simulink model "pfb_coeff_sim"  (R2016b)
settings: Solver=VariableStepAuto  StartTime=0.0  StopTime=8192*0.5  RelTol=1e-3
undefined symbols (not defined in the file): fft_stages
libraries: xbsIndex_r4 x6420, casper_library_misc x5, casper_library_sources x4, xps_library x1, casper_library_delays x1
(part 18 of 36)

== system pfb_coeff_sim/pfb/pfb_fir_generic/pfb_fir_coeff_gen ==
  sync : Inport
  din : Inport  Port=2
  en : Inport  Port=3
  a_expand : Subsystem  AncestorBlock=casper_library_flow_control/bus_expand  mask(bus_expand){mode=divisions of equal size, outputNum=64, outputWidth=18, outputBinaryPt=0, outputArithmeticType=0, show_format=off, outputToWorkspace=off, variablePrefix=out, outputToModelAsWell=on}
      mask prompts: outputNum "Number of outputs:"; outputWidth "Output width:"; outputBinaryPt "Output binary point position:"; outputArithmeticType "Output arithmetic type (ufix=0, fix=1, bool=2):"; show_format "Print format string?"; outputToWorkspace "Output to workspace?"; variablePrefix "Variable name prefix:"; outputToModelAsWell "Output to model as well?"
      mask help:
      | Expands a 'bus' made using a bus_create or Xilinx
      | concat block.
      | The input will be divided into the specified number
      | of outputs with the specified arithmetic types.
      | Divisions are made from most significant bit.
      mask init: same as pfb_coeff_sim/bus_expand5
      settings: AttributesFormatString=64 outputs
      mask TypeOptions mode: divisions of equal size | divisions of arbitrary size
      mask Callback mode: bus_expand_callback();
      mask Callback outputWidth: bus_expand_callback();
      mask Callback outputToWorkspace: bus_expand_callback();
  b_expand : Subsystem  AncestorBlock=casper_library_flow_control/bus_expand  mask(bus_expand){mode=divisions of equal size, outputNum=64, outputWidth=18, outputBinaryPt=0, outputArithmeticType=0, show_format=off, outputToWorkspace=off, variablePrefix=out, outputToModelAsWell=on}
      mask prompts: outputNum "Number of outputs:"; outputWidth "Output width:"; outputBinaryPt "Output binary point position:"; outputArithmeticType "Output arithmetic type (ufix=0, fix=1, bool=2):"; show_format "Print format string?"; outputToWorkspace "Output to workspace?"; variablePrefix "Variable name prefix:"; outputToModelAsWell "Output to model as well?"
      mask help:
      | Expands a 'bus' made using a bus_create or Xilinx
      | concat block.
      | The input will be divided into the specified number
      | of outputs with the specified arithmetic types.
      | Divisions are made from most significant bit.
      mask init: same as pfb_coeff_sim/bus_expand5
      settings: AttributesFormatString=64 outputs
      mask TypeOptions mode: divisions of equal size | divisions of arbitrary size
      mask Callback mode: bus_expand_callback();
      mask Callback outputWidth: bus_expand_callback();
      mask Callback outputToWorkspace: bus_expand_callback();
  concat : xbsIndex_r4/Concat  num_inputs=128  dbl_ovrd=off  block_type=concat
  const0 : xbsIndex_r4/Constant  const=1  gui_display_data_type=Fixed-point  arith_type=Signed (2's comp)  n_bits=18  bin_pt=17  preci_type=Single  exp_width=8  frac_width=24  explicit_period=on  period=1  equ=P=C  opselect=C  inp2=PCIN>>17  opr=+  inp1=P  carry=CIN  dbl_ovrd=off  block_type=constant
  const1 : xbsIndex_r4/Constant  const=3.7497e-17  gui_display_data_type=Fixed-point  arith_type=Signed (2's comp)  n_bits=18  bin_pt=17  preci_type=Single  exp_width=8  frac_width=24  explicit_period=on  period=1  equ=P=C  opselect=C  inp2=PCIN>>17  opr=+  inp1=P  carry=CIN  dbl_ovrd=off  block_type=constant
  const2 : xbsIndex_r4/Constant  const=-3.3271e-17  gui_display_data_type=Fixed-point  arith_type=Signed (2's comp)  n_bits=18  bin_pt=17  preci_type=Single  exp_width=8  frac_width=24  explicit_period=on  period=1  equ=P=C  opselect=C  inp2=PCIN>>17  opr=+  inp1=P  carry=CIN  dbl_ovrd=off  block_type=constant
  const3 : xbsIndex_r4/Constant  const=2.6947e-17  gui_display_data_type=Fixed-point  arith_type=Signed (2's comp)  n_bits=18  bin_pt=17  preci_type=Single  exp_width=8  frac_width=24  explicit_period=on  period=1  equ=P=C  opselect=C  inp2=PCIN>>17  opr=+  inp1=P  carry=CIN  dbl_ovrd=off  block_type=constant
  const4 : xbsIndex_r4/Constant  const=-1.9488e-17  gui_display_data_type=Fixed-point  arith_type=Signed (2's comp)  n_bits=18  bin_pt=17  preci_type=Single  exp_width=8  frac_width=24  explicit_period=on  period=1  equ=P=C  opselect=C  inp2=PCIN>>17  opr=+  inp1=P  carry=CIN  dbl_ovrd=off  block_type=constant
  const5 : xbsIndex_r4/Constant  const=1.2029e-17  gui_display_data_type=Fixed-point  arith_type=Signed (2's comp)  n_bits=18  bin_pt=17  preci_type=Single  exp_width=8  frac_width=24  explicit_period=on  period=1  equ=P=C  opselect=C  inp2=PCIN>>17  opr=+  inp1=P  carry=CIN  dbl_ovrd=off  block_type=constant
  const6 : xbsIndex_r4/Constant  const=-5.7064e-18  gui_display_data_type=Fixed-point  arith_type=Signed (2's comp)  n_bits=18  bin_pt=17  preci_type=Single  exp_width=8  frac_width=24  explicit_period=on  period=1  equ=P=C  opselect=C  inp2=PCIN>>17  opr=+  inp1=P  carry=CIN  dbl_ovrd=off  block_type=constant
  const7 : xbsIndex_r4/Constant  const=1.4823e-18  gui_display_data_type=Fixed-point  arith_type=Signed (2's comp)  n_bits=18  bin_pt=17  preci_type=Single  exp_width=8  frac_width=24  explicit_period=on  period=1  equ=P=C  opselect=C  inp2=PCIN>>17  opr=+  inp1=P  carry=CIN  dbl_ovrd=off  block_type=constant
  counter : xbsIndex_r4/Counter  cnt_type=Free Running  cnt_to=Inf  operation=Up  start_count=0  cnt_by_val=1  arith_type=Unsigned  n_bits=8  bin_pt=0  load_pin=off  rst=on  en=on  explicit_period=on  period=1  use_behavioral_HDL=off  implementation=Fabric  dbl_ovrd=off  block_type=counter
  d{0..63,65..71,73..79,81..87,89..95,97..103,105..111,113..119,121..127} (120 alike) : xbsIndex_r4/Delay  rst=off  infoeditControl=Selection of Reset will increase slice count due to use of real FFs and instead of SRLs  en=off  latency=1  reg_retiming=on  dbl_ovrd=off  block_type=delay
      settings: infoedit=Hardware notes: A delay line is a chain, each link of which is an SRL16 or SRL32 followed by a flip-flop.
  d{64,72,80,88,96,104,112,120} (8 alike) : xbsIndex_r4/Delay  rst=off  infoeditControl=Selection of Reset will increase slice count due to use of real FFs and instead of SRLs  en=on  latency=1  reg_retiming=on  dbl_ovrd=off  block_type=delay
      settings: infoedit=Hardware notes: A delay line is a chain, each link of which is an SRL16 or SRL32 followed by a flip-flop.
  den0 : xbsIndex_r4/Delay  rst=off  infoeditControl=Selection of Reset will increase slice count due to use of real FFs and instead of SRLs  en=off  latency=9  reg_retiming=on  dbl_ovrd=off  block_type=delay
      settings: infoedit=Hardware notes: A delay line is a chain, each link of which is an SRL16 or SRL32 followed by a flip-flop.
  den1 : xbsIndex_r4/Delay  rst=off  infoeditControl=Selection of Reset will increase slice count due to use of real FFs and instead of SRLs  en=off  latency=1  reg_retiming=on  dbl_ovrd=off  block_type=delay
      settings: infoedit=Hardware notes: A delay line is a chain, each link of which is an SRL16 or SRL32 followed by a flip-flop.
  dfirst : xbsIndex_r4/Delay  rst=off  infoeditControl=Selection of Reset will increase slice count due to use of real FFs and instead of SRLs  en=off  latency=3  reg_retiming=on  dbl_ovrd=off  block_type=delay
      settings: infoedit=Hardware notes: A delay line is a chain, each link of which is an SRL16 or SRL32 followed by a flip-flop.
  din_delay : xbsIndex_r4/Delay  rst=off  infoeditControl=Selection of Reset will increase slice count due to use of real FFs and instead of SRLs  en=off  latency=10  reg_retiming=on  dbl_ovrd=off  block_type=delay
      settings: infoedit=Hardware notes: A delay line is a chain, each link of which is an SRL16 or SRL32 followed by a flip-flop.
  first : xbsIndex_r4/Relational  mode=a=b  op_type=Bool  en=off  latency=6  dbl_ovrd=off  block_type=relational
  inverter : xbsIndex_r4/Inverter  en=off  latency=0  dbl_ovrd=off  block_type=inv
  munge : Subsystem  AncestorBlock=casper_library_flow_control/munge  mask(munge){divisions=64, div_size=[18 18 18 18 18 18 18 18 18 18 18 18 18 18 18 18 18 18 18 18 18 18 18 18 18 18 18 18 18 18 18 18 18 18 18 18 18 18 18 18 18 18 18 18 18 18 18 18 18 18 18 18 18 18 18 18 18 18 18 18 18 18 18 18], order=[56 63 62 61 60 59 58 57 48 55 54 53 52 51 50 49 40 47 46 45 44 43 42 41 32 39 38 37 36 35 34 33 24 31 30 29 28 27 26 25 16 23 22 21 20 19 18 17 8 15 14 13 12 11 10 9 0 7 6 5 4 3 2 1], arith_type_out=Unsigned, bin_pt_out=0}
      mask prompts: divisions "Number of divisions"; div_size "Division size (bits)"; order "Division packing order"; arith_type_out "Output arithmetic type"; bin_pt_out "Output binary point"
      mask help: Splits an input bus into the specified number of divisions and then recombines them in the order specified (most significant division = 0,least = number divisions-1)
      mask init:
      | munge_init(gcb, ...
      |     'divisions', divisions, ...
      |     'div_size', div_size, ...
      |     'order', order, ...
      |     'arith_type_out', arith_type_out, ...
      |     'bin_pt_out', bin_pt_out);
      settings: AttributesFormatString=|
      | split:[18 18 18 18 18 18 18 18 18 18 18 18 18 18 18 18 18 18 18 18 18 18 18 18 18 18 18 18 18 18 18 18 18 18 18 18 18 18 18 18 18 18 18 18 18 18 18 18 18 18 18 18 18 18 18 18 18 18 18 18 18 18 18 18]
      | join:[56 63 62 61 60 59 58 57 48 55 54 53 52 51 50 49 40 47 46 45 44 43 42 41 32 39 38 37 36 35 34 33 24 31 30 29 28 27 26 25 16 23 22 21 20 19 18 17 8 15 14 13 12 11 10 9 0 7 6 5 4 3 2 1]
      | Unsigned [1152,0]
      mask TypeOptions arith_type_out: Unsigned | Signed  (2's comp) | Floating-point
  mux{0..7} (8 alike) : xbsIndex_r4/Mux  inputs=2  en=off  latency=1  precision=Full  arith_type=Unsigned  n_bits=16  bin_pt=14  quantization=Truncate  overflow=Wrap  dbl_ovrd=off  block_type=mux
  reinterpret{0..7} (8 alike) : xbsIndex_r4/Reinterpret  force_arith_type=on  arith_type=Unsigned  force_bin_pt=on  bin_pt=0  block_type=reinterpret
  rom : Subsystem  AncestorBlock=casper_library_bus/bus_dual_port_ram  mask(bus_dual_port_ram){n_bits=[18 18 18 18 18 18 18 18 18 18 18 18 18 18 18 18 18 18 18 18 18 18 18 18 18 18 18 18 18 18 18 18 18 18 18 18 18 18 18 18 18 18 18 18 18 18 18 18 18 18 18 18 18 18 18 18 18 18 18 18 18 18 18 18], bin_pts=[17 17 17 17 17 17 17 17 17 17 17 17 17 17 17 17 17 17 17 17 17 17 17 17 17 17 17 17 17 17 17 17 17 17 17 17 17 17 17 17 17 17 17 17 17 17 17 17 17 17 17 17 17 17 17 17 17 17 17 17 17 17 17 17], init_vector=[pfb_coeff_gen_calc(11, 16, 'hann', 3, 0, 1, 1, false)', pfb_coeff_gen_calc(11, 16, 'hann', 3, 1, 1, 1, false)', pfb_coeff_gen_calc(11, 16, 'hann', 3, 2, 1, 1, false)', pfb_coeff_gen_calc(11, 16, 'hann', 3, 3, 1, 1, false)', pfb_coeff_gen_calc(11, 16, 'hann', 3, 4, 1, 1, false)', pfb_coeff_gen_calc(11, 16, 'hann', 3, 5, 1, 1, false)', pfb_coeff_gen_calc(11, 16, 'hann', 3, 6, 1, 1, false)', pfb_coeff_gen_calc(11, 16, 'hann', 3, 7, 1, 1, false)', pfb_coeff_gen_calc(11, 16, 'hann', 3, 0, 1, 2, false)', pfb_coeff_gen_calc(11, 16, 'hann', 3, 1, 1, 2, false)', pfb_coeff_gen_calc(11, 16, 'hann', 3, 2, 1, 2, false)', pfb_coeff_gen_calc(11, 16, 'hann', 3, 3, 1, 2, false)', pfb_coeff_gen_calc(11, 16, 'hann', 3, 4, 1, 2, false)', pfb_coeff_gen_calc(11, 16, 'hann', 3, 5, 1, 2, false)', pfb_coeff_gen_calc(11, 16, 'hann', 3, 6, 1, 2, false)', pfb_coeff_gen_calc(11, 16, 'hann', 3, 7, 1, 2, false)', pfb_coeff_gen_calc(11, 16, 'hann', 3, 0, 1, 3, false)', pfb_coeff_gen_calc(11, 16, 'hann', 3, 1, 1, 3, false)', pfb_coeff_gen_calc(11, 16, 'hann', 3, 2, 1, 3, false)', pfb_coeff_gen_calc(11, 16, 'hann', 3, 3, 1, 3, false)', pfb_coeff_gen_calc(11, 16, 'hann', 3, 4, 1, 3, false)', pfb_coeff_gen_calc(11, 16, 'hann', 3, 5, 1, 3, false)', pfb_coeff_gen_calc(11, 16, 'hann', 3, 6, 1, 3, false)', pfb_coeff_gen_calc(11, 16, 'hann', 3, 7, 1, 3, false)', pfb_coeff_gen_calc(11, 16, 'hann', 3, 0, 1, 4, false)', pfb_coeff_gen_calc(11, 16, 'hann', 3, 1, 1, 4, false)', pfb_coeff_gen_calc(11, 16, 'hann', 3, 2, 1, 4, false)', pfb_coeff_gen_calc(11, 16, 'hann', 3, 3, 1, 4, false)', pfb_coeff_gen_calc(11, 16, 'hann', 3, 4, 1, 4, false)', pfb_coeff_gen_calc(11, 16, 'hann', 3, 5, 1, 4, false)', pfb_coeff_gen_calc(11, 16, 'hann', 3, 6, 1, 4, false)', pfb_coeff_gen_calc(11, 16, 'hann', 3, 7, 1, 4, false)', pfb_coeff_gen_calc(11, 16, 'hann', 3, 0, 1, 5, false)', pfb_coeff_gen_calc(11, 16, 'hann', 3, 1, 1, 5, false)', pfb_coeff_gen_calc(11, 16, 'hann', 3, 2, 1, 5, false)', pfb_coeff_gen_calc(11, 16, 'hann', 3, 3, 1, 5, false)', pfb_coeff_gen_calc(11, 16, 'hann', 3, 4, 1, 5, false)', pfb_coeff_gen_calc(11, 16, 'hann', 3, 5, 1, 5, false)', pfb_coeff_gen_calc(11, 16, 'hann', 3, 6, 1, 5, false)', pfb_coeff_gen_calc(11, 16, 'hann', 3, 7, 1, 5, false)', pfb_coeff_gen_calc(11, 16, 'hann', 3, 0, 1, 6, false)', pfb_coeff_gen_calc(11, 16, 'hann', 3, 1, 1, 6, false)', pfb_coeff_gen_calc(11, 16, 'hann', 3, 2, 1, 6, false)', pfb_coeff_gen_calc(11, 16, 'hann', 3, 3, 1, 6, false)', pfb_coeff_gen_calc(11, 16, 'hann', 3, 4, 1, 6, false)', pfb_coeff_gen_calc(11, 16, 'hann', 3, 5, 1, 6, false)', pfb_coeff_gen_calc(11, 16, 'hann', 3, 6, 1, 6, false)', pfb_coeff_gen_calc(11, 16, 'hann', 3, 7, 1, 6, false)', pfb_coeff_gen_calc(11, 16, 'hann', 3, 0, 1, 7, false)', pfb_coeff_gen_calc(11, 16, 'hann', 3, 1, 1, 7, false)', pfb_coeff_gen_calc(11, 16, 'hann', 3, 2, 1, 7, false)', pfb_coeff_gen_calc(11, 16, 'hann', 3, 3, 1, 7, false)', pfb_coeff_gen_calc(11, 16, 'hann', 3, 4, 1, 7, false)', pfb_coeff_gen_calc(11, 16, 'hann', 3, 5, 1, 7, false)', pfb_coeff_gen_calc(11, 16, 'hann', 3, 6, 1, 7, false)', pfb_coeff_gen_calc(11, 16, 'hann', 3, 7, 1, 7, false)', pfb_coeff_gen_calc(11, 16, 'hann', 3, 0, 1, 8, false)', pfb_coeff_gen_calc(11, 16, 'hann', 3, 1, 1, 8, false)', pfb_coeff_gen_calc(11, 16, 'hann', 3, 2, 1, 8, false)', pfb_coeff_gen_calc(11, 16, 'hann', 3, 3, 1, 8, false)', pfb_coeff_gen_calc(11, 16, 'hann', 3, 4, 1, 8, false)', pfb_coeff_gen_calc(11, 16, 'hann', 3, 5, 1, 8, false)', pfb_coeff_gen_calc(11, 16, 'hann', 3, 6, 1, 8, false)', pfb_coeff_gen_calc(11, 16, 'hann', 3, 7, 1, 8, false)'], max_fanout=1, mem_type=Block RAM, bram_optimization=Speed, async_a=off, async_b=off, b_to_a_ratio_bits=0, misc=off, bram_latency=3, fan_latency=6, addra_register=on, addra_implementation=core, dina_register=off, dina_implementation=behavioral, wea_register=off, wea_implementation=behavioral, ena_register=off, ena_implementation=core, addrb_register=on, addrb_implementation=core, dinb_register=off, dinb_implementation=behavioral, web_register=off, web_implementation=behavioral, enb_register=off, enb_implementation=core}
      mask prompts: n_bits "data word bit widths"; bin_pts "data word binary points"; init_vector "initial value vector"; max_fanout "limit fanout to ?"; mem_type "memory type"; bram_optimization "memory optimization"; async_a "a asynchronous"; async_b "b asynchronous"; b_to_a_ratio_bits "b_to_a ratio bits"; misc "misc support"; bram_latency "bram latency"; fan_latency "input register latency"; addra_register "addra input register"; addra_implementation "addra register implementation"; dina_register "dina input register"; dina_implementation "dina register implementation"; wea_register "wea input register"; wea_implementation "wea register implementation"; ena_register "ena input register"; ena_implementation "ena register implementation"; addrb_register "addrb input register"; addrb_implementation "addrb register implementation"; dinb_register "dinb input register"; dinb_implementation "dinb register implementation"; web_register "web input register"; web_implementation "web register implementation"; enb_register "enb input register"; enb_implementation "enb register implementation"
      mask help: RAM for a bus allowing fanout control
      mask init:
      | bus_dual_port_ram_init(gcb, ...
      |     'n_bits', n_bits, ...
      |     'bin_pts', bin_pts, ...
      |     'init_vector', init_vector, ...
      |     'max_fanout', max_fanout, ...
      |     'mem_type', mem_type, ...
      |     'bram_optimization', bram_optimization, ...
      |     'async_a', async_a, ...
      |     'async_b', async_b, ...
      |     'b_to_a_ratio_bits', b_to_a_ratio_bits, ...
      |     'misc', misc, ...
      |     'bram_latency', bram_latency, ...
      |     'fan_latency', fan_latency, ...
      |     'addra_register', addra_register, ...
      |     'addra_implementation', addra_implementation, ...
      |     'dina_register', dina_register, ...
      |     'dina_implementation', dina_implementation, ...
      |     'wea_register', wea_register, ...
      |     'wea_implementation', wea_implementation, ...
      |     'ena_register', ena_register, ...
      |     'ena_implementation', ena_implementation, ...
      |     'addrb_register', addrb_register, ...
      |     'addrb_implementation', addrb_implementation, ...
      |     'dinb_register', dinb_register, ...
      |     'dinb_implementation', dinb_implementation, ...
      |     'web_register', web_register, ...
      |     'web_implementation', web_implementation, ...
      |     'enb_register', enb_register, ...
      |     'enb_implementation', enb_implementation);
      mask TypeOptions mem_type: Distributed memory | Block RAM
      mask TypeOptions bram_optimization: Area | Speed
      mask TypeOptions addra_implementation: core | behavioral
      mask TypeOptions dina_implementation: core | behavioral
      mask TypeOptions wea_implementation: core | behavioral
      mask TypeOptions ena_implementation: core | behavioral
      mask TypeOptions addrb_implementation: core | behavioral
      mask TypeOptions dinb_implementation: core | behavioral
      mask TypeOptions web_implementation: core | behavioral
      mask TypeOptions enb_implementation: core | behavioral
  rom_din : xbsIndex_r4/Constant  const=0  gui_display_data_type=Fixed-point  arith_type=Unsigned  n_bits=1152  bin_pt=0  preci_type=Single  exp_width=8  frac_width=24  explicit_period=on  period=1  equ=P=C  opselect=C  inp2=PCIN>>17  opr=+  inp1=P  carry=CIN  dbl_ovrd=off  block_type=constant
  rom_we : xbsIndex_r4/Constant  const=0  gui_display_data_type=Fixed-point  arith_type=Boolean  n_bits=16  bin_pt=14  preci_type=Single  exp_width=8  frac_width=24  explicit_period=on  period=1  equ=P=C  opselect=C  inp2=PCIN>>17  opr=+  inp1=P  carry=CIN  dbl_ovrd=off  block_type=constant
  sync_delay : xbsIndex_r4/Delay  rst=off  infoeditControl=Selection of Reset will increase slice count due to use of real FFs and instead of SRLs  en=off  latency=10  reg_retiming=on  dbl_ovrd=off  block_type=delay
      settings: infoedit=Hardware notes: A delay line is a chain, each link of which is an SRL16 or SRL32 followed by a flip-flop.
  zero : xbsIndex_r4/Constant  const=0  gui_display_data_type=Fixed-point  arith_type=Unsigned  n_bits=8  bin_pt=0  preci_type=Single  exp_width=8  frac_width=24  explicit_period=on  period=1  equ=P=C  opselect=C  inp2=PCIN>>17  opr=+  inp1=P  carry=CIN  dbl_ovrd=off  block_type=constant
  sync_out : Outport
  dout : Outport  Port=2
  coeffs : Outport  Port=3
  dvalid : Outport  Port=4
  wires:
  sync/1 -> sync_delay/1, counter/1
  sync_delay/1 -> sync_out/1
  din/1 -> din_delay/1
  din_delay/1 -> dout/1
  counter/1 -> inverter/1, rom/1(addra), first/2
  inverter/1 -> rom/4(addrb)
  rom_din/1 -> rom/2(dina), rom/5(dinb)
  rom_we/1 -> rom/3(wea), rom/6(web)
  zero/1 -> first/1
  first/1 -> dfirst/1
  rom/2(B) -> munge/1(din)
  rom/1(A) -> a_expand/1(bus_in)
  munge/1(dout) -> b_expand/1(bus_in)
  concat/1 -> coeffs/1
  a_expand/1(msb_out64) -> d0/1
  d0/1 -> concat/1
  a_expand/2(out63) -> d1/1
  d1/1 -> concat/2
  a_expand/3(out62) -> d2/1
  d2/1 -> concat/3
  a_expand/4(out61) -> d3/1
  d3/1 -> concat/4
  a_expand/5(out60) -> d4/1
  d4/1 -> concat/5
  a_expand/6(out59) -> d5/1
  d5/1 -> concat/6
  a_expand/7(out58) -> d6/1
  d6/1 -> concat/7
  a_expand/8(out57) -> d7/1
  d7/1 -> concat/8
  a_expand/9(out56) -> d8/1
  d8/1 -> concat/9
  a_expand/10(out55) -> d9/1
  d9/1 -> concat/10
  a_expand/11(out54) -> d10/1
  d10/1 -> concat/11
  a_expand/12(out53) -> d11/1
  d11/1 -> concat/12
  a_expand/13(out52) -> d12/1
  d12/1 -> concat/13
  a_expand/14(out51) -> d13/1
  d13/1 -> concat/14
  a_expand/15(out50) -> d14/1
  d14/1 -> concat/15
  a_expand/16(out49) -> d15/1
  d15/1 -> concat/16
  a_expand/17(out48) -> d16/1
  d16/1 -> concat/17
  a_expand/18(out47) -> d17/1
  d17/1 -> concat/18
  a_expand/19(out46) -> d18/1
  d18/1 -> concat/19
  a_expand/20(out45) -> d19/1
  d19/1 -> concat/20
  a_expand/21(out44) -> d20/1
  d20/1 -> concat/21
  a_expand/22(out43) -> d21/1
  d21/1 -> concat/22
  a_expand/23(out42) -> d22/1
  d22/1 -> concat/23
  a_expand/24(out41) -> d23/1
  d23/1 -> concat/24
  a_expand/25(out40) -> d24/1
  d24/1 -> concat/25
  a_expand/26(out39) -> d25/1
  d25/1 -> concat/26
  a_expand/27(out38) -> d26/1
  d26/1 -> concat/27
  a_expand/28(out37) -> d27/1
  d27/1 -> concat/28
  a_expand/29(out36) -> d28/1
  d28/1 -> concat/29
  a_expand/30(out35) -> d29/1
  d29/1 -> concat/30
  a_expand/31(out34) -> d30/1
  d30/1 -> concat/31
  a_expand/32(out33) -> d31/1
  d31/1 -> concat/32
  a_expand/33(out32) -> d32/1
  d32/1 -> concat/33
  a_expand/34(out31) -> d33/1
  d33/1 -> concat/34
  a_expand/35(out30) -> d34/1
  d34/1 -> concat/35
  a_expand/36(out29) -> d35/1
  d35/1 -> concat/36
  a_expand/37(out28) -> d36/1
  d36/1 -> concat/37
  a_expand/38(out27) -> d37/1
  d37/1 -> concat/38
  a_expand/39(out26) -> d38/1
  d38/1 -> concat/39
  a_expand/40(out25) -> d39/1
  d39/1 -> concat/40
  a_expand/41(out24) -> d40/1
  d40/1 -> concat/41
  a_expand/42(out23) -> d41/1
  d41/1 -> concat/42
  a_expand/43(out22) -> d42/1
  d42/1 -> concat/43
  a_expand/44(out21) -> d43/1
  d43/1 -> concat/44
  a_expand/45(out20) -> d44/1
  d44/1 -> concat/45
  a_expand/46(out19) -> d45/1
  d45/1 -> concat/46
  a_expand/47(out18) -> d46/1
  d46/1 -> concat/47
  a_expand/48(out17) -> d47/1
  d47/1 -> concat/48
  a_expand/49(out16) -> d48/1
  d48/1 -> concat/49
  a_expand/50(out15) -> d49/1
  d49/1 -> concat/50
  a_expand/51(out14) -> d50/1
  d50/1 -> concat/51
  a_expand/52(out13) -> d51/1
  d51/1 -> concat/52
  a_expand/53(out12) -> d52/1
  d52/1 -> concat/53
  a_expand/54(out11) -> d53/1
  d53/1 -> concat/54
  a_expand/55(out10) -> d54/1
  d54/1 -> concat/55
  a_expand/56(out9) -> d55/1
  d55/1 -> concat/56
  a_expand/57(out8) -> d56/1
  d56/1 -> concat/57
  a_expand/58(out7) -> d57/1
  d57/1 -> concat/58
  a_expand/59(out6) -> d58/1
  d58/1 -> concat/59
  a_expand/60(out5) -> d59/1
  d59/1 -> concat/60
  a_expand/61(out4) -> d60/1
  d60/1 -> concat/61
  a_expand/62(out3) -> d61/1
  d61/1 -> concat/62
  a_expand/63(out2) -> d62/1
  d62/1 -> concat/63
  a_expand/64(lsb_out1) -> d63/1
  d63/1 -> concat/64
  b_expand/1(msb_out64) -> d64/1
  const0/1 -> reinterpret0/1
  reinterpret0/1 -> mux0/3
  dfirst/1 -> mux0/1, mux1/1, mux2/1, mux3/1, mux4/1, mux5/1, mux6/1, mux7/1
  d64/1 -> mux0/2
  mux0/1 -> concat/65
  b_expand/2(out63) -> d65/1
  d65/1 -> concat/66
  b_expand/3(out62) -> d66/1
  d66/1 -> concat/67
  b_expand/4(out61) -> d67/1
  d67/1 -> concat/68
  b_expand/5(out60) -> d68/1
  d68/1 -> concat/69
  b_expand/6(out59) -> d69/1
  d69/1 -> concat/70
  b_expand/7(out58) -> d70/1
  d70/1 -> concat/71
  b_expand/8(out57) -> d71/1
  d71/1 -> concat/72
  b_expand/9(out56) -> d72/1
  const1/1 -> reinterpret1/1
  reinterpret1/1 -> mux1/3
  d72/1 -> mux1/2
  mux1/1 -> concat/73
  b_expand/10(out55) -> d73/1
  d73/1 -> concat/74
  b_expand/11(out54) -> d74/1
  d74/1 -> concat/75
  b_expand/12(out53) -> d75/1
  d75/1 -> concat/76
  b_expand/13(out52) -> d76/1
  d76/1 -> concat/77
  b_expand/14(out51) -> d77/1
  d77/1 -> concat/78
  b_expand/15(out50) -> d78/1
  d78/1 -> concat/79
  b_expand/16(out49) -> d79/1
  d79/1 -> concat/80
  b_expand/17(out48) -> d80/1
  const2/1 -> reinterpret2/1
  reinterpret2/1 -> mux2/3
  d80/1 -> mux2/2
  mux2/1 -> concat/81
  b_expand/18(out47) -> d81/1
  d81/1 -> concat/82
  b_expand/19(out46) -> d82/1
  d82/1 -> concat/83
  b_expand/20(out45) -> d83/1
  d83/1 -> concat/84
  b_expand/21(out44) -> d84/1
  d84/1 -> concat/85
  b_expand/22(out43) -> d85/1
  d85/1 -> concat/86
  b_expand/23(out42) -> d86/1
  d86/1 -> concat/87
  b_expand/24(out41) -> d87/1
  d87/1 -> concat/88
  b_expand/25(out40) -> d88/1
  const3/1 -> reinterpret3/1
  reinterpret3/1 -> mux3/3
  d88/1 -> mux3/2
  mux3/1 -> concat/89
  b_expand/26(out39) -> d89/1
  d89/1 -> concat/90
  b_expand/27(out38) -> d90/1
  d90/1 -> concat/91
  b_expand/28(out37) -> d91/1
  d91/1 -> concat/92
  b_expand/29(out36) -> d92/1
  d92/1 -> concat/93
  b_expand/30(out35) -> d93/1
  d93/1 -> concat/94
  b_expand/31(out34) -> d94/1
  d94/1 -> concat/95
  b_expand/32(out33) -> d95/1
  d95/1 -> concat/96
  b_expand/33(out32) -> d96/1
  const4/1 -> reinterpret4/1
  reinterpret4/1 -> mux4/3
  d96/1 -> mux4/2
  mux4/1 -> concat/97
  b_expand/34(out31) -> d97/1
  d97/1 -> concat/98
  b_expand/35(out30) -> d98/1
  d98/1 -> concat/99
  b_expand/36(out29) -> d99/1
  d99/1 -> concat/100
  b_expand/37(out28) -> d100/1
  d100/1 -> concat/101
  b_expand/38(out27) -> d101/1
  d101/1 -> concat/102
  b_expand/39(out26) -> d102/1
  d102/1 -> concat/103
  b_expand/40(out25) -> d103/1
  d103/1 -> concat/104
  b_expand/41(out24) -> d104/1
  const5/1 -> reinterpret5/1
  reinterpret5/1 -> mux5/3
  d104/1 -> mux5/2
  mux5/1 -> concat/105
  b_expand/42(out23) -> d105/1
  d105/1 -> concat/106
  b_expand/43(out22) -> d106/1
  d106/1 -> concat/107
  b_expand/44(out21) -> d107/1
  d107/1 -> concat/108
  b_expand/45(out20) -> d108/1
  d108/1 -> concat/109
  b_expand/46(out19) -> d109/1
  d109/1 -> concat/110
  b_expand/47(out18) -> d110/1
  d110/1 -> concat/111
  b_expand/48(out17) -> d111/1
  d111/1 -> concat/112
  b_expand/49(out16) -> d112/1
  const6/1 -> reinterpret6/1
  reinterpret6/1 -> mux6/3
  d112/1 -> mux6/2
  mux6/1 -> concat/113
  b_expand/50(out15) -> d113/1
  d113/1 -> concat/114
  b_expand/51(out14) -> d114/1
  d114/1 -> concat/115
  b_expand/52(out13) -> d115/1
  d115/1 -> concat/116
  b_expand/53(out12) -> d116/1
  d116/1 -> concat/117
  b_expand/54(out11) -> d117/1
  d117/1 -> concat/118
  b_expand/55(out10) -> d118/1
  d118/1 -> concat/119
  b_expand/56(out9) -> d119/1
  d119/1 -> concat/120
  b_expand/57(out8) -> d120/1
  const7/1 -> reinterpret7/1
  reinterpret7/1 -> mux7/3
  d120/1 -> mux7/2
  mux7/1 -> concat/121
  b_expand/58(out7) -> d121/1
  d121/1 -> concat/122
  b_expand/59(out6) -> d122/1
  d122/1 -> concat/123
  b_expand/60(out5) -> d123/1
  d123/1 -> concat/124
  b_expand/61(out4) -> d124/1
  d124/1 -> concat/125
  b_expand/62(out3) -> d125/1
  d125/1 -> concat/126
  b_expand/63(out2) -> d126/1
  d126/1 -> concat/127
  b_expand/64(lsb_out1) -> d127/1
  d127/1 -> concat/128
  en/1 -> counter/2, den0/1
  den0/1 -> d64/2, d72/2, d80/2, d88/2, d96/2, d104/2, d112/2, d120/2, den1/1
  den1/1 -> dvalid/1

== system pfb_coeff_sim/pfb/pfb_fir_generic/pfb_fir_taps ==
  sync : Inport
  din : Inport  Port=2
  coeffs : Inport  Port=3
  en : Inport  Port=4
  arnold : Terminator
  bram_din : xbsIndex_r4/Concat  num_inputs=2  dbl_ovrd=off  block_type=concat
  bus_adder_tree : Subsystem  AncestorBlock=casper_library_bus/bus_adder_tree  mask(bus_adder_tree){n_busses=16, n_bits=[28 28 28 28 28 28 28 28], bin_pts=26, dtypes=1, add_latency=4, first_stage_hdl=on, adder_imp=Behavioral, misc=off}
      mask prompts: n_busses "number of busses"; n_bits "bus component bit widths"; bin_pts "bus component binary points"; dtypes "bus component data types"; add_latency "adder latency"; first_stage_hdl "implement first stage in of adders in behavioral HDL?"; adder_imp "adder implementation"; misc "misc support"
      mask help: Add components of multiple identical busses
      mask init:
      | bus_adder_tree_init(gcb, ...
      |     'n_busses', n_busses, ...
      |     'n_bits', n_bits, ...
      |     'bin_pts', bin_pts, ...
      |     'dtypes', dtypes, ...
      |     'add_latency', add_latency, ...
      |     'first_stage_hdl', first_stage_hdl, ...
      |     'adder_imp', adder_imp, ...
      |     'misc', misc);
      mask TypeOptions adder_imp: Behavioral | Fabric | DSP48
  bus_mult : Subsystem  AncestorBlock=casper_library_bus/bus_mult  mask(bus_mult){n_bits_a=[10 10 10 10 10 10 10 10 10 10 10 10 10 10 10 10 10 10 10 10 10 10 10 10 10 10 10 10 10 10 10 10 10 10 10 10 10 10 10 10 10 10 10 10 10 10 10 10 10 10 10 10 10 10 10 10 10 10 10 10 10 10 10 10 10 10 10 10 10 10 10 10 10 10 10 10 10 10 10 10 10 10 10 10 10 10 10 10 10 10 10 10 10 10 10 10 10 10 10 10 10 10 10 10 10 10 10 10 10 10 10 10 10 10 10 10 10 10 10 10 10 10 10 10 10 10 10 10], bin_pt_a=9, type_a=1, cmplx_a=off, n_bits_b=[18 18 18 18 18 18 18 18 18 18 18 18 18 18 18 18 18 18 18 18 18 18 18 18 18 18 18 18 18 18 18 18 18 18 18 18 18 18 18 18 18 18 18 18 18 18 18 18 18 18 18 18 18 18 18 18 18 18 18 18 18 18 18 18 18 18 18 18 18 18 18 18 18 18 18 18 18 18 18 18 18 18 18 18 18 18 18 18 18 18 18 18 18 18 18 18 18 18 18 18 18 18 18 18 18 18 18 18 18 18 18 18 18 18 18 18 18 18 18 18 18 18 18 18 18 18 18 18], bin_pt_b=17, type_b=1, cmplx_b=off, misc=off, floating_point=off, float_type=single, input_vec_a=1, input_vec_b=1, frac_width=19, exp_width=6, n_bits_out=n_bits_data+n_bits_coeff, bin_pt_out=n_bits_data-1+bin_pt_coeff, type_out=1, quantization=0, overflow=0, mult_latency=mult_latency, add_latency=0, conv_latency=0, max_fanout=1, fan_latency=0, multiplier_implementation=behavioral HDL, pipeline_cmult_en=off, pipeline_latency=0}
      mask prompts: n_bits_a "a input bit widths"; bin_pt_a "a input binary points"; type_a "a input type (Unsigned=0, Signed=1)"; cmplx_a "a input complex"; n_bits_b "b input bit widths"; bin_pt_b "b input binary points"; type_b "b input type (Unsigned=0, Signed=1)"; cmplx_b "b input complex"; misc "misc support"; floating_point "floating point"; float_type "float type"; input_vec_a "a input vector in bus"; input_vec_b "b input vector in bus"; frac_width "fraction width"; exp_width "exponent width"; n_bits_out "output bit widths"; bin_pt_out "output binary points"; type_out "output type (Unsigned=0, Signed=1)"; quantization "quantization strategy (Truncate=0, Round  (unbiased: +/- Inf)=1)"; overflow "overflow strategy (Wrap=0, Saturate=1, Flag as error=2)"; mult_latency "multiplier latency"; add_latency "adder latency"; conv_latency "convert latency"; max_fanout "limit fanout to ?"; fan_latency "fanout register latency"; multiplier_implementation "multiplier implementation"; pipeline_cmult_en "pipeline complex mult"; pipeline_latency "pipeline latency"
      mask help: Multiply components of two busses
      mask init:
      | bus_mult_init(gcb, ...
      |     'n_bits_a', n_bits_a, ...
      |     'bin_pt_a', bin_pt_a, ...
      |     'type_a', type_a, ...
      |     'cmplx_a', cmplx_a, ...
      |     'n_bits_b', n_bits_b, ...
      |     'bin_pt_b', bin_pt_b, ...
      |     'type_b', type_b, ...
      |     'cmplx_b', cmplx_b, ...
      |     'n_bits_out', n_bits_out, ...
      |     'bin_pt_out', bin_pt_out, ...
      |     'type_out', type_out, ...
      |     'floating_point', floating_point, ...
      |     'float_type', float_type, ...
      |     'exp_width', exp_width, ...
      |     'input_vec_a', input_vec_a, ...
      |     'input_vec_b', input_vec_b, ...
      |     'frac_width', frac_width, ...         
      |     'quantization', quantization, ...
      |     'overflow', overflow, ...
      |     'mult_latency', mult_latency, ...
      |     'add_latency', add_latency, ...
      |     'conv_latency', conv_latency, ...
      |     'max_fanout', max_fanout, ...
      |     'pipeline_cmult_en', pipeline_cmult_en, ...
      |     'pipeline_latency', pipeline_latency, ...
      |     'fan_latency', fan_latency, ...
      |     'multiplier_implementation', multiplier_implementation, ...
      |     'misc', misc);
      mask Callback floating_point:
      | onoff = get_param(gcb, 'floating_point');
      | if strcmp(onoff,'on')
      |     enable_fixpt = 'off'
      |     set_param_state(gcb, 'float_type', 'on')
      | 
      |     set_param_state(gcb, 'input_vec_a', 'on')
      |     set_param_state(gcb, 'input_vec_b', 'on')
      | 
      |     f_type = get_param(gcb, 'float_type')
      |     if strcmp(f_type,'custom')
      |         set_param_state(gcb, 'exp_width', 'on')
      |         set_param_state(gcb, 'frac_width', 'on')
      |     else
      |         set_param_state(gcb, 'exp_width', 'off')
      |         set_param_state(gcb, 'frac_width', 'off')
      |     end
      | 
      | else
      |     enable_fixpt = 'on'
      |     set_param_state(gcb, 'float_type', 'off')
      |     set_param_state(gcb, 'exp_width', 'off')
      |     set_param_state(gcb, 'frac_width', 'off')
      |     set_param_state(gcb, 'input_vec_a', 'off')
      |     set_param_state(gcb, 'input_vec_b', 'off')
      | end
      | 
      | set_param_state(gcb, 'n_bits_a', enable_fixpt)
      | set_param_state(gcb, 'bin_pt_a', enable_fixpt)
      | set_param_state(gcb, 'type_a', enable_fixpt)
      | set_param_state(gcb, 'n_bits_b', enable_fixpt)
      | set_param_state(gcb, 'bin_pt_b', enable_fixpt)
      | set_param_state(gcb, 'type_b', enable_fixpt)
      | 
      | set_param_state(gcb, 'n_bits_out', enable_fixpt)
      | set_param_state(gcb, 'bin_pt_out', enable_fixpt)
      | set_param_state(gcb, 'type_out', enable_fixpt)
      | set_param_state(gcb, 'quantization', enable_fixpt)
      | set_param_state(gcb, 'overflow', enable_fixpt)
      mask TypeOptions float_type: single | custom
      mask Callback float_type:
      | f_type = get_param(gcb, 'float_type')
      | if strcmp(f_type,'custom')
      |     set_param_state(gcb, 'exp_width', 'on')
      |     set_param_state(gcb, 'frac_width', 'on')
      | else
      |     set_param_state(gcb, 'exp_width', 'off')
      |     set_param_state(gcb, 'frac_width', 'off')
      | end
      mask TypeOptions multiplier_implementation: behavioral HDL | standard core | embedded multiplier core
      mask Callback pipeline_cmult_en:
      | pipeline_en = get_param(gcb, 'pipeline_cmult_en');
      | if strcmp(pipeline_en,'on')
      | 
      |     set_param_state(gcb, 'pipeline_latency', 'on')
      | else
      |     set_param_state(gcb, 'pipeline_latency', 'off')
      | end
  counter : xbsIndex_r4/Counter  cnt_type=Free Running  cnt_to=Inf  operation=Up  start_count=0  cnt_by_val=1  arith_type=Unsigned  n_bits=8  bin_pt=0  load_pin=off  rst=on  en=on  explicit_period=on  period=1  use_behavioral_HDL=off  implementation=Fabric  dbl_ovrd=off  block_type=counter
  daddr : xbsIndex_r4/Delay  rst=off  infoeditControl=Selection of Reset will increase slice count due to use of real FFs and instead of SRLs  en=off  latency=9  reg_retiming=on  dbl_ovrd=off  block_type=delay
      settings: infoedit=Hardware notes: A delay line is a chain, each link of which is an SRL16 or SRL32 followed by a flip-flop.
  dcoeffs : xbsIndex_r4/Delay  rst=off  infoeditControl=Selection of Reset will increase slice count due to use of real FFs and instead of SRLs  en=off  latency=9  reg_retiming=on  dbl_ovrd=off  block_type=delay
      settings: infoedit=Hardware notes: A delay line is a chain, each link of which is an SRL16 or SRL32 followed by a flip-flop.
  ddin : xbsIndex_r4/Delay  rst=off  infoeditControl=Selection of Reset will increase slice count due to use of real FFs and instead of SRLs  en=off  latency=9  reg_retiming=off  dbl_ovrd=off  block_type=delay
      settings: infoedit=Hardware notes: A delay line is a chain, each link of which is an SRL16 or SRL32 followed by a flip-flop.
  den0 : xbsIndex_r4/Delay  rst=off  infoeditControl=Selection of Reset will increase slice count due to use of real FFs and instead of SRLs  en=off  latency=9  reg_retiming=on  dbl_ovrd=off  block_type=delay
      settings: infoedit=Hardware notes: A delay line is a chain, each link of which is an SRL16 or SRL32 followed by a flip-flop.
  den1 : xbsIndex_r4/Delay  rst=off  infoeditControl=Selection of Reset will increase slice count due to use of real FFs and instead of SRLs  en=off  latency=3  reg_retiming=on  dbl_ovrd=off  block_type=delay
      settings: infoedit=Hardware notes: A delay line is a chain, each link of which is an SRL16 or SRL32 followed by a flip-flop.
  den2 : xbsIndex_r4/Delay  rst=off  infoeditControl=Selection of Reset will increase slice count due to use of real FFs and instead of SRLs  en=off  latency=16  reg_retiming=on  dbl_ovrd=off  block_type=delay
      settings: infoedit=Hardware notes: A delay line is a chain, each link of which is an SRL16 or SRL32 followed by a flip-flop.
  dsync0 : xbsIndex_r4/Delay  rst=off  infoeditControl=Selection of Reset will increase slice count due to use of real FFs and instead of SRLs  en=off  latency=9  reg_retiming=on  dbl_ovrd=off  block_type=delay
      settings: infoedit=Hardware notes: A delay line is a chain, each link of which is an SRL16 or SRL32 followed by a flip-flop.
  dsync1 : xbsIndex_r4/Delay  rst=off  infoeditControl=Selection of Reset will increase slice count due to use of real FFs and instead of SRLs  en=off  latency=3  reg_retiming=on  dbl_ovrd=off  block_type=delay
      settings: infoedit=Hardware notes: A delay line is a chain, each link of which is an SRL16 or SRL32 followed by a flip-flop.
  dsync2 : xbsIndex_r4/Delay  rst=off  infoeditControl=Selection of Reset will increase slice count due to use of real FFs and instead of SRLs  en=off  latency=16  reg_retiming=on  dbl_ovrd=off  block_type=delay
      settings: infoedit=Hardware notes: A delay line is a chain, each link of which is an SRL16 or SRL32 followed by a flip-flop.
  mult_din : xbsIndex_r4/Concat  num_inputs=2  dbl_ovrd=off  block_type=concat
  never : xbsIndex_r4/Constant  const=0  gui_display_data_type=Fixed-point  arith_type=Boolean  n_bits=16  bin_pt=14  preci_type=Single  exp_width=8  frac_width=24  explicit_period=on  period=1  equ=P=C  opselect=C  inp2=PCIN>>17  opr=+  inp1=P  carry=CIN  dbl_ovrd=off  block_type=constant
  sync_delay : casper_library_delays/sync_delay_en  DelayLen=(2^(pfb_size-n_inputs))*(n_taps-1)
  tap_delays : Subsystem  AncestorBlock=casper_library_bus/bus_dual_port_ram  mask(bus_dual_port_ram){n_bits=[10 10 10 10 10 10 10 10 10 10 10 10 10 10 10 10 10 10 10 10 10 10 10 10 10 10 10 10 10 10 10 10 10 10 10 10 10 10 10 10 10 10 10 10 10 10 10 10 10 10 10 10 10 10 10 10 10 10 10 10 10 10 10 10 10 10 10 10 10 10 10 10 10 10 10 10 10 10 10 10 10 10 10 10 10 10 10 10 10 10 10 10 10 10 10 10 10 10 10 10 10 10 10 10 10 10 10 10 10 10 10 10 10 10 10 10 10 10 10 10], bin_pts=[0 0 0 0 0 0 0 0 0 0 0 0 0 0 0 0 0 0 0 0 0 0 0 0 0 0 0 0 0 0 0 0 0 0 0 0 0 0 0 0 0 0 0 0 0 0 0 0 0 0 0 0 0 0 0 0 0 0 0 0 0 0 0 0 0 0 0 0 0 0 0 0 0 0 0 0 0 0 0 0 0 0 0 0 0 0 0 0 0 0 0 0 0 0 0 0 0 0 0 0 0 0 0 0 0 0 0 0 0 0 0 0 0 0 0 0 0 0 0 0], init_vector=repmat(zeros(256, 1), 1, 120), max_fanout=1, mem_type=Block RAM, bram_optimization=Speed, async_a=off, async_b=off, b_to_a_ratio_bits=0, misc=off, bram_latency=3, fan_latency=6, addra_register=on, addra_implementation=core, dina_register=off, dina_implementation=behavioral, wea_register=off, wea_implementation=behavioral, ena_register=off, ena_implementation=behavioral, addrb_register=on, addrb_implementation=core, dinb_register=on, dinb_implementation=core, web_register=on, web_implementation=core, enb_register=off, enb_implementation=behavioral}
      mask prompts: n_bits "data word bit widths"; bin_pts "data word binary points"; init_vector "initial value vector"; max_fanout "limit fanout to ?"; mem_type "memory type"; bram_optimization "memory optimization"; async_a "a asynchronous"; async_b "b asynchronous"; b_to_a_ratio_bits "b_to_a ratio bits"; misc "misc support"; bram_latency "bram latency"; fan_latency "input register latency"; addra_register "addra input register"; addra_implementation "addra register implementation"; dina_register "dina input register"; dina_implementation "dina register implementation"; wea_register "wea input register"; wea_implementation "wea register implementation"; ena_register "ena input register"; ena_implementation "ena register implementation"; addrb_register "addrb input register"; addrb_implementation "addrb register implementation"; dinb_register "dinb input register"; dinb_implementation "dinb register implementation"; web_register "web input register"; web_implementation "web register implementation"; enb_register "enb input register"; enb_implementation "enb register implementation"
      mask help: RAM for a bus allowing fanout control
      mask init: same as pfb_coeff_sim/pfb/pfb_fir_generic/pfb_fir_coeff_gen/rom
      mask TypeOptions mem_type: Distributed memory | Block RAM
      mask TypeOptions bram_optimization: Area | Speed
      mask TypeOptions addra_implementation: core | behavioral
      mask TypeOptions dina_implementation: core | behavioral
      mask TypeOptions wea_implementation: core | behavioral
      mask TypeOptions ena_implementation: core | behavioral
      mask TypeOptions addrb_implementation: core | behavioral
      mask TypeOptions dinb_implementation: core | behavioral
      mask TypeOptions web_implementation: core | behavioral
      mask TypeOptions enb_implementation: core | behavioral
  tap_split : Subsystem  AncestorBlock=casper_library_flow_control/bus_expand  mask(bus_expand){mode=divisions of equal size, outputNum=16, outputWidth=224, outputBinaryPt=0, outputArithmeticType=0, show_format=off, outputToWorkspace=off, variablePrefix=out, outputToModelAsWell=on}
      mask prompts: outputNum "Number of outputs:"; outputWidth "Output width:"; outputBinaryPt "Output binary point position:"; outputArithmeticType "Output arithmetic type (ufix=0, fix=1, bool=2):"; show_format "Print format string?"; outputToWorkspace "Output to workspace?"; variablePrefix "Variable name prefix:"; outputToModelAsWell "Output to model as well?"
      mask help:
      | Expands a 'bus' made using a bus_create or Xilinx
      | concat block.
      | The input will be divided into the specified number
      | of outputs with the specified arithmetic types.
      | Divisions are made from most significant bit.
      mask init: same as pfb_coeff_sim/bus_expand5
      settings: AttributesFormatString=16 outputs
      mask TypeOptions mode: divisions of equal size | divisions of arbitrary size
      mask Callback mode: bus_expand_callback();
      mask Callback outputWidth: bus_expand_callback();
      mask Callback outputToWorkspace: bus_expand_callback();
  youngest : xbsIndex_r4/Slice  nbits=(1*n_bits_data)*(n_taps-2)*(2^n_inputs)*n_streams  boolean_output=off  mode=Upper Bit Location + Width  bit1=0  base1=MSB of Input  bit0=0  base0=LSB of Input  dbl_ovrd=off  block_type=slice
  sync_out : Outport
  dout : Outport  Port=2
  dvalid : Outport  Port=3
  wires:
  dsync0/1 -> dsync1/1
  dsync1/1 -> dsync2/1
  dsync2/1 -> sync_out/1
  din/1 -> ddin/1
  coeffs/1 -> dcoeffs/1
  en/1 -> den0/1, sync_delay/2, counter/2
  den0/1 -> den1/1, tap_delays/6(web)
  den1/1 -> den2/1
  sync/1 -> sync_delay/1, counter/1
  sync_delay/1 -> dsync0/1
  ddin/1 -> bram_din/1, mult_din/1
  youngest/1 -> bram_din/2
  counter/1 -> daddr/1, tap_delays/1(addra)
  bram_din/1 -> tap_delays/2(dina), tap_delays/5(dinb)
  never/1 -> tap_delays/3(wea)
  daddr/1 -> tap_delays/4(addrb)
  tap_delays/2(B) -> arnold/1
  tap_delays/1(A) -> mult_din/2, youngest/1
  mult_din/1 -> bus_mult/1(a)
  dcoeffs/1 -> bus_mult/2(b)
  bus_mult/1(a*b) -> tap_split/1(bus_in)
  tap_split/1(msb_out16) -> bus_adder_tree/1(d0)
  tap_split/2(out15) -> bus_adder_tree/2(d1)
  tap_split/3(out14) -> bus_adder_tree/3(d2)
  tap_split/4(out13) -> bus_adder_tree/4(d3)
  tap_split/5(out12) -> bus_adder_tree/5(d4)
  tap_split/6(out11) -> bus_adder_tree/6(d5)
  tap_split/7(out10) -> bus_adder_tree/7(d6)
  tap_split/8(out9) -> bus_adder_tree/8(d7)
  tap_split/9(out8) -> bus_adder_tree/9(d8)
  tap_split/10(out7) -> bus_adder_tree/10(d9)
  tap_split/11(out6) -> bus_adder_tree/11(d10)
  tap_split/12(out5) -> bus_adder_tree/12(d11)
  tap_split/13(out4) -> bus_adder_tree/13(d12)
  tap_split/14(out3) -> bus_adder_tree/14(d13)
  tap_split/15(out2) -> bus_adder_tree/15(d14)
  tap_split/16(lsb_out1) -> bus_adder_tree/16(d15)
  bus_adder_tree/1(out) -> dout/1
  den2/1 -> dvalid/1

== system pfb_coeff_sim/pfb/pfb_fir_generic/tap_split1 ==
  bus_in : Inport
  reinterpret1 : xbsIndex_r4/Reinterpret  force_arith_type=on  arith_type=Unsigned  force_bin_pt=on  bin_pt=0  block_type=reinterpret
  reinterpret2 : xbsIndex_r4/Reinterpret  force_arith_type=on  arith_type=Unsigned  force_bin_pt=on  bin_pt=0  block_type=reinterpret
  slice1 : xbsIndex_r4/Slice  nbits=1152  boolean_output=off  mode=Upper Bit Location + Width  bit1=-1152  base1=MSB of Input  bit0=0  base0=LSB of Input  dbl_ovrd=off  block_type=slice
  slice2 : xbsIndex_r4/Slice  nbits=1152  boolean_output=off  mode=Upper Bit Location + Width  bit1=0  base1=MSB of Input  bit0=0  base0=LSB of Input  dbl_ovrd=off  block_type=slice
  msb_out2 : Outport
  lsb_out1 : Outport  Port=2
  wires:
  bus_in/1 -> slice2/1, slice1/1
  slice2/1 -> reinterpret2/1
  reinterpret2/1 -> msb_out2/1
  slice1/1 -> reinterpret1/1
  reinterpret1/1 -> lsb_out1/1
